simulink model "gm_uz_pmsm_model_9ph_vnl"  (R2021b)
settings: Solver=FixedStepAuto  StartTime=0.0  StopTime=0.8  RelTol=1e-3
PreLoadFcn:
  | uz_pmsm_model_9ph_init_parameter
undefined symbols (not defined in the file or in its folder): a, b, c, friction_coefficient, inertia, k_i_d, k_i_q, k_p_d, k_p_q, Kpd, L_d, L_o1, L_o2, L_q, L_x1, L_x2, L_y1, L_y2, L_zero, polepair, psi_pm, R_1, static_friction_torque, Tnd, ts
libraries: hdlmdlgenlib x191, hdlsllib x90, dspsigops x19, simulink x17, slpidlib x2, spsAlphaBetaZerotodq0Lib x1, pid_lib x1, spsdq0toAlphaBetaZeroLib x1
(part 7 of 7)

== system gm_uz_pmsm_model_9ph_vnl/uz_pmsm_model_9ph/Transformation1/Divide ==
  In1 : Inport
  In2 : Inport  Port=2
  Divide : Product  Inputs=**  OutDataTypeStr=single  SampleTime=1e-08
  Divide_pd1 : Delay  DelayLength=6
  Out1 : Outport
  wires:
  Divide_pd1/1 -> Out1/1
  Divide/1 -> Divide_pd1/1
  In2/1 -> Divide/2
  In1/1 -> Divide/1

== system gm_uz_pmsm_model_9ph_vnl/uz_pmsm_model_9ph/Transformation1/Divide1 ==
  In1 : Inport
  In2 : Inport  Port=2
  Divide1 : Product  Inputs=**  OutDataTypeStr=single  SampleTime=1e-08
  Divide1_pd1 : Delay  DelayLength=6
  Out1 : Outport
  wires:
  Divide1_pd1/1 -> Out1/1
  Divide1/1 -> Divide1_pd1/1
  In2/1 -> Divide1/2
  In1/1 -> Divide1/1

== system gm_uz_pmsm_model_9ph_vnl/uz_pmsm_model_9ph/Transformation1/Divide2 ==
  In1 : Inport
  In2 : Inport  Port=2
  Divide2 : Product  Inputs=**  OutDataTypeStr=single  SampleTime=1e-08
  Divide2_pd1 : Delay  DelayLength=6
  Out1 : Outport
  wires:
  Divide2_pd1/1 -> Out1/1
  Divide2/1 -> Divide2_pd1/1
  In2/1 -> Divide2/2
  In1/1 -> Divide2/1

== system gm_uz_pmsm_model_9ph_vnl/uz_pmsm_model_9ph/Transformation1/Divide3 ==
  In1 : Inport
  In2 : Inport  Port=2
  Divide3 : Product  Inputs=**  OutDataTypeStr=single  SampleTime=1e-08
  Divide3_pd1 : Delay  DelayLength=6
  Out1 : Outport
  wires:
  Divide3_pd1/1 -> Out1/1
  Divide3/1 -> Divide3_pd1/1
  In2/1 -> Divide3/2
  In1/1 -> Divide3/1

== system gm_uz_pmsm_model_9ph_vnl/uz_pmsm_model_9ph/Transformation1/Transformation1_MAC ==
  in0 : Inport  OutDataTypeStr=fixdt(1, 18, 16)  PortDimensions=[9 1]  SampleTime=1e-08
  in1 : Inport  Port=2  OutDataTypeStr=fixdt(1, 25, 12)  PortDimensions=[9]  SampleTime=1e-08
  globalSchedule : EnablePort  OutDataTypeStr=boolean
  PipelineRegister : Delay  DelayLength=double(8)  InitialCondition=0
  t : hdlsllib/HDL Operations/Multiply-Accumulate  opMode=Vector  initValueSetting=Dialog  initValue=0  initValueSetting2=Dialog  initValue2=0  initValueSetting3=Dialog  initValue3=0  num_samples=2  RndMeth2=Floor  RndMeth3=Floor  OutDataTypeStr=fixdt(1, 43, 28)  datatype2=Inherit: Inherit via back propagation  datatype3=Inherit: Inherit via back propagation  validOut=on  endInandOut=on  startOut=on  countOut=on  dim=-1  DoSatur=off  parallel=off
      settings: SourceProductBaseCode=SL
  out0 : Outport  OutDataTypeStr=fixdt(1, 43, 28)  SampleTime=1e-08  InitialOutput=0
  wires:
  t/1 -> PipelineRegister/1
  in1/1 -> t/2
  in0/1 -> t/1
  PipelineRegister/1 -> out0/1

== system gm_uz_pmsm_model_9ph_vnl/uz_pmsm_model_9ph/Transformation1/Transformation1_MAC1 ==
  in0 : Inport  OutDataTypeStr=fixdt(1, 18, 16)  PortDimensions=[9 1]  SampleTime=1e-08
  in1 : Inport  Port=2  OutDataTypeStr=fixdt(1, 25, 12)  PortDimensions=[9]  SampleTime=1e-08
  globalSchedule : EnablePort  OutDataTypeStr=boolean
  PipelineRegister : Delay  DelayLength=double(8)  InitialCondition=0
  t : hdlsllib/HDL Operations/Multiply-Accumulate  opMode=Vector  initValueSetting=Dialog  initValue=0  initValueSetting2=Dialog  initValue2=0  initValueSetting3=Dialog  initValue3=0  num_samples=2  RndMeth2=Floor  RndMeth3=Floor  OutDataTypeStr=fixdt(1, 43, 28)  datatype2=Inherit: Inherit via back propagation  datatype3=Inherit: Inherit via back propagation  validOut=on  endInandOut=on  startOut=on  countOut=on  dim=-1  DoSatur=off  parallel=off
      settings: SourceProductBaseCode=SL
  out0 : Outport  OutDataTypeStr=fixdt(1, 43, 28)  SampleTime=1e-08  InitialOutput=0
  wires:
  t/1 -> PipelineRegister/1
  in1/1 -> t/2
  in0/1 -> t/1
  PipelineRegister/1 -> out0/1

== system gm_uz_pmsm_model_9ph_vnl/uz_pmsm_model_9ph/Transformation1/Transformation1_MAC2 ==
  in0 : Inport  OutDataTypeStr=fixdt(1, 18, 16)  PortDimensions=[9 1]  SampleTime=1e-08
  in1 : Inport  Port=2  OutDataTypeStr=fixdt(1, 25, 12)  PortDimensions=[9]  SampleTime=1e-08
  globalSchedule : EnablePort  OutDataTypeStr=boolean
  PipelineRegister : Delay  DelayLength=double(8)  InitialCondition=0
  t : hdlsllib/HDL Operations/Multiply-Accumulate  opMode=Vector  initValueSetting=Dialog  initValue=0  initValueSetting2=Dialog  initValue2=0  initValueSetting3=Dialog  initValue3=0  num_samples=2  RndMeth2=Floor  RndMeth3=Floor  OutDataTypeStr=fixdt(1, 43, 28)  datatype2=Inherit: Inherit via back propagation  datatype3=Inherit: Inherit via back propagation  validOut=on  endInandOut=on  startOut=on  countOut=on  dim=-1  DoSatur=off  parallel=off
      settings: SourceProductBaseCode=SL
  out0 : Outport  OutDataTypeStr=fixdt(1, 43, 28)  SampleTime=1e-08  InitialOutput=0
  wires:
  t/1 -> PipelineRegister/1
  in1/1 -> t/2
  in0/1 -> t/1
  PipelineRegister/1 -> out0/1

== system gm_uz_pmsm_model_9ph_vnl/uz_pmsm_model_9ph/Transformation1/Transformation1_MAC3 ==
  in0 : Inport  OutDataTypeStr=fixdt(1, 18, 16)  PortDimensions=[9 1]  SampleTime=1e-08
  in1 : Inport  Port=2  OutDataTypeStr=fixdt(1, 25, 12)  PortDimensions=[9]  SampleTime=1e-08
  globalSchedule : EnablePort  OutDataTypeStr=boolean
  PipelineRegister : Delay  DelayLength=double(8)  InitialCondition=0
  t : hdlsllib/HDL Operations/Multiply-Accumulate  opMode=Vector  initValueSetting=Dialog  initValue=0  initValueSetting2=Dialog  initValue2=0  initValueSetting3=Dialog  initValue3=0  num_samples=2  RndMeth2=Floor  RndMeth3=Floor  OutDataTypeStr=fixdt(1, 43, 28)  datatype2=Inherit: Inherit via back propagation  datatype3=Inherit: Inherit via back propagation  validOut=on  endInandOut=on  startOut=on  countOut=on  dim=-1  DoSatur=off  parallel=off
      settings: SourceProductBaseCode=SL
  out0 : Outport  OutDataTypeStr=fixdt(1, 43, 28)  SampleTime=1e-08  InitialOutput=0
  wires:
  t/1 -> PipelineRegister/1
  in1/1 -> t/2
  in0/1 -> t/1
  PipelineRegister/1 -> out0/1

== system gm_uz_pmsm_model_9ph_vnl/uz_pmsm_model_9ph/Transformation1/Transformation1_MAC4 ==
  in0 : Inport  OutDataTypeStr=fixdt(1, 18, 16)  PortDimensions=[9 1]  SampleTime=1e-08
  in1 : Inport  Port=2  OutDataTypeStr=fixdt(1, 25, 12)  PortDimensions=[9]  SampleTime=1e-08
  globalSchedule : EnablePort  OutDataTypeStr=boolean
  PipelineRegister : Delay  DelayLength=double(8)  InitialCondition=0
  t : hdlsllib/HDL Operations/Multiply-Accumulate  opMode=Vector  initValueSetting=Dialog  initValue=0  initValueSetting2=Dialog  initValue2=0  initValueSetting3=Dialog  initValue3=0  num_samples=2  RndMeth2=Floor  RndMeth3=Floor  OutDataTypeStr=fixdt(1, 43, 28)  datatype2=Inherit: Inherit via back propagation  datatype3=Inherit: Inherit via back propagation  validOut=on  endInandOut=on  startOut=on  countOut=on  dim=-1  DoSatur=off  parallel=off
      settings: SourceProductBaseCode=SL
  out0 : Outport  OutDataTypeStr=fixdt(1, 43, 28)  SampleTime=1e-08  InitialOutput=0
  wires:
  t/1 -> PipelineRegister/1
  in1/1 -> t/2
  in0/1 -> t/1
  PipelineRegister/1 -> out0/1

== system gm_uz_pmsm_model_9ph_vnl/uz_pmsm_model_9ph/Transformation1/Transformation1_MAC5 ==
  in0 : Inport  OutDataTypeStr=fixdt(1, 18, 16)  PortDimensions=[9 1]  SampleTime=1e-08
  in1 : Inport  Port=2  OutDataTypeStr=fixdt(1, 25, 12)  PortDimensions=[9]  SampleTime=1e-08
  globalSchedule : EnablePort  OutDataTypeStr=boolean
  PipelineRegister : Delay  DelayLength=double(8)  InitialCondition=0
  t : hdlsllib/HDL Operations/Multiply-Accumulate  opMode=Vector  initValueSetting=Dialog  initValue=0  initValueSetting2=Dialog  initValue2=0  initValueSetting3=Dialog  initValue3=0  num_samples=2  RndMeth2=Floor  RndMeth3=Floor  OutDataTypeStr=fixdt(1, 43, 28)  datatype2=Inherit: Inherit via back propagation  datatype3=Inherit: Inherit via back propagation  validOut=on  endInandOut=on  startOut=on  countOut=on  dim=-1  DoSatur=off  parallel=off
      settings: SourceProductBaseCode=SL
  out0 : Outport  OutDataTypeStr=fixdt(1, 43, 28)  SampleTime=1e-08  InitialOutput=0
  wires:
  t/1 -> PipelineRegister/1
  in1/1 -> t/2
  in0/1 -> t/1
  PipelineRegister/1 -> out0/1

== system gm_uz_pmsm_model_9ph_vnl/uz_pmsm_model_9ph/Transformation1/Transformation1_MAC6 ==
  in0 : Inport  OutDataTypeStr=fixdt(1, 18, 16)  PortDimensions=[9 1]  SampleTime=1e-08
  in1 : Inport  Port=2  OutDataTypeStr=fixdt(1, 25, 12)  PortDimensions=[9]  SampleTime=1e-08
  globalSchedule : EnablePort  OutDataTypeStr=boolean
  PipelineRegister : Delay  DelayLength=double(8)  InitialCondition=0
  t : hdlsllib/HDL Operations/Multiply-Accumulate  opMode=Vector  initValueSetting=Dialog  initValue=0  initValueSetting2=Dialog  initValue2=0  initValueSetting3=Dialog  initValue3=0  num_samples=2  RndMeth2=Floor  RndMeth3=Floor  OutDataTypeStr=fixdt(1, 43, 28)  datatype2=Inherit: Inherit via back propagation  datatype3=Inherit: Inherit via back propagation  validOut=on  endInandOut=on  startOut=on  countOut=on  dim=-1  DoSatur=off  parallel=off
      settings: SourceProductBaseCode=SL
  out0 : Outport  OutDataTypeStr=fixdt(1, 43, 28)  SampleTime=1e-08  InitialOutput=0
  wires:
  t/1 -> PipelineRegister/1
  in1/1 -> t/2
  in0/1 -> t/1
  PipelineRegister/1 -> out0/1

== system gm_uz_pmsm_model_9ph_vnl/uz_pmsm_model_9ph/Transformation1/Transformation1_MAC7 ==
  in0 : Inport  OutDataTypeStr=fixdt(1, 18, 16)  PortDimensions=[9 1]  SampleTime=1e-08
  in1 : Inport  Port=2  OutDataTypeStr=fixdt(1, 25, 12)  PortDimensions=[9]  SampleTime=1e-08
  globalSchedule : EnablePort  OutDataTypeStr=boolean
  PipelineRegister : Delay  DelayLength=double(8)  InitialCondition=0
  t : hdlsllib/HDL Operations/Multiply-Accumulate  opMode=Vector  initValueSetting=Dialog  initValue=0  initValueSetting2=Dialog  initValue2=0  initValueSetting3=Dialog  initValue3=0  num_samples=2  RndMeth2=Floor  RndMeth3=Floor  OutDataTypeStr=fixdt(1, 43, 28)  datatype2=Inherit: Inherit via back propagation  datatype3=Inherit: Inherit via back propagation  validOut=on  endInandOut=on  startOut=on  countOut=on  dim=-1  DoSatur=off  parallel=off
      settings: SourceProductBaseCode=SL
  out0 : Outport  OutDataTypeStr=fixdt(1, 43, 28)  SampleTime=1e-08  InitialOutput=0
  wires:
  t/1 -> PipelineRegister/1
  in1/1 -> t/2
  in0/1 -> t/1
  PipelineRegister/1 -> out0/1

== system gm_uz_pmsm_model_9ph_vnl/uz_pmsm_model_9ph/Transformation1/Transformation1_MAC8 ==
  in0 : Inport  OutDataTypeStr=fixdt(1, 18, 16)  PortDimensions=[9 1]  SampleTime=1e-08
  in1 : Inport  Port=2  OutDataTypeStr=fixdt(1, 25, 12)  PortDimensions=[9]  SampleTime=1e-08
  globalSchedule : EnablePort  OutDataTypeStr=boolean
  PipelineRegister : Delay  DelayLength=double(8)  InitialCondition=0
  t : hdlsllib/HDL Operations/Multiply-Accumulate  opMode=Vector  initValueSetting=Dialog  initValue=0  initValueSetting2=Dialog  initValue2=0  initValueSetting3=Dialog  initValue3=0  num_samples=2  RndMeth2=Floor  RndMeth3=Floor  OutDataTypeStr=fixdt(1, 43, 28)  datatype2=Inherit: Inherit via back propagation  datatype3=Inherit: Inherit via back propagation  validOut=on  endInandOut=on  startOut=on  countOut=on  dim=-1  DoSatur=off  parallel=off
      settings: SourceProductBaseCode=SL
  out0 : Outport  OutDataTypeStr=fixdt(1, 43, 28)  SampleTime=1e-08  InitialOutput=0
  wires:
  t/1 -> PipelineRegister/1
  in1/1 -> t/2
  in0/1 -> t/1
  PipelineRegister/1 -> out0/1

== system gm_uz_pmsm_model_9ph_vnl/uz_pmsm_model_9ph/Transformation1/t3 ==
  in0 : Inport
  ColVec1 : Selector  NumberOfDimensions=2  IndexOptions=Select all,Index vector (dialog)  Indices=1,1  OutputSizes=1,1
  ColVec2 : Selector  NumberOfDimensions=2  IndexOptions=Select all,Index vector (dialog)  Indices=1,2  OutputSizes=1,1
  ColVec3 : Selector  NumberOfDimensions=2  IndexOptions=Select all,Index vector (dialog)  Indices=1,3  OutputSizes=1,1
  ColVec4 : Selector  NumberOfDimensions=2  IndexOptions=Select all,Index vector (dialog)  Indices=1,4  OutputSizes=1,1
  ColVec5 : Selector  NumberOfDimensions=2  IndexOptions=Select all,Index vector (dialog)  Indices=1,5  OutputSizes=1,1
  ColVec6 : Selector  NumberOfDimensions=2  IndexOptions=Select all,Index vector (dialog)  Indices=1,6  OutputSizes=1,1
  ColVec7 : Selector  NumberOfDimensions=2  IndexOptions=Select all,Index vector (dialog)  Indices=1,7  OutputSizes=1,1
  ColVec8 : Selector  NumberOfDimensions=2  IndexOptions=Select all,Index vector (dialog)  Indices=1,8  OutputSizes=1,1
  ColVec9 : Selector  NumberOfDimensions=2  IndexOptions=Select all,Index vector (dialog)  Indices=1,9  OutputSizes=1,1
  out0 : Outport
  out1 : Outport  Port=2
  out2 : Outport  Port=3
  out3 : Outport  Port=4
  out4 : Outport  Port=5
  out5 : Outport  Port=6
  out6 : Outport  Port=7
  out7 : Outport  Port=8
  out8 : Outport  Port=9
  wires:
  ColVec9/1 -> out8/1
  ColVec8/1 -> out7/1
  ColVec7/1 -> out6/1
  ColVec6/1 -> out5/1
  ColVec5/1 -> out4/1
  ColVec4/1 -> out3/1
  ColVec3/1 -> out2/1
  ColVec2/1 -> out1/1
  ColVec1/1 -> out0/1
  in0/1 -> ColVec9/1, ColVec8/1, ColVec7/1, ColVec6/1, ColVec5/1, ColVec4/1, ColVec3/1, ColVec2/1, ColVec1/1

== system gm_uz_pmsm_model_9ph_vnl/uz_pmsm_model_9ph/Wrapped State DTI/Compare To Constant1_relop ==
  In1 : Inport
  In2 : Inport  Port=2
  Compare To Constant1_relop : RelationalOperator  Operator=<  OutDataTypeStr=boolean  SampleTime=1e-08  RndMeth=Nearest  InputSameDT=on
  Compare To Constant1_relop_pd1 : Delay  DelayLength=1
  Out1 : Outport
  wires:
  Compare To Constant1_relop_pd1/1 -> Out1/1
  Compare To Constant1_relop/1 -> Compare To Constant1_relop_pd1/1
  In2/1 -> Compare To Constant1_relop/2
  In1/1 -> Compare To Constant1_relop/1

== system gm_uz_pmsm_model_9ph_vnl/uz_pmsm_model_9ph/Wrapped State DTI/Compare To Constant_relop ==
  In1 : Inport
  In2 : Inport  Port=2
  Compare To Constant_relop : RelationalOperator  OutDataTypeStr=boolean  SampleTime=1e-08  RndMeth=Nearest  InputSameDT=on
  Compare To Constant_relop_pd1 : Delay  DelayLength=1
  Out1 : Outport
  wires:
  Compare To Constant_relop_pd1/1 -> Out1/1
  Compare To Constant_relop/1 -> Compare To Constant_relop_pd1/1
  In2/1 -> Compare To Constant_relop/2
  In1/1 -> Compare To Constant_relop/1

== system gm_uz_pmsm_model_9ph_vnl/uz_pmsm_model_9ph/Wrapped State DTI/Gain ==
  In1 : Inport
  In2 : Inport  Port=2
  Gain : Product  Inputs=**  OutDataTypeStr=single  SampleTime=1e-08
  Gain_pd1 : Delay  DelayLength=6
  Out1 : Outport
  wires:
  Gain_pd1/1 -> Out1/1
  Gain/1 -> Gain_pd1/1
  In2/1 -> Gain/2
  In1/1 -> Gain/1

== system gm_uz_pmsm_model_9ph_vnl/uz_pmsm_model_9ph/Wrapped State DTI/Product ==
  In1 : Inport
  In2 : Inport  Port=2
  Product : Product  Inputs=**  OutDataTypeStr=single  SampleTime=1e-08
  Product_pd1 : Delay  DelayLength=6
  Out1 : Outport
  wires:
  Product_pd1/1 -> Out1/1
  Product/1 -> Product_pd1/1
  In2/1 -> Product/2
  In1/1 -> Product/1

== system gm_uz_pmsm_model_9ph_vnl/uz_pmsm_model_9ph/Wrapped State DTI/Sum ==
  In1 : Inport
  In2 : Inport  Port=2
  Sum : Sum  OutDataTypeStr=single  SampleTime=1e-08
  Sum_pd1 : Delay  DelayLength=6
  Out1 : Outport
  wires:
  Sum_pd1/1 -> Out1/1
  Sum/1 -> Sum_pd1/1
  In2/1 -> Sum/2
  In1/1 -> Sum/1

== system gm_uz_pmsm_model_9ph_vnl/uz_pmsm_model_9ph/Wrapped State DTI/Sum1 ==
  In1 : Inport
  In2 : Inport  Port=2
  Sum1 : Sum  Inputs=+-  OutDataTypeStr=single  SampleTime=1e-08
  Sum1_pd1 : Delay  DelayLength=6
  Out1 : Outport
  wires:
  Sum1_pd1/1 -> Out1/1
  Sum1/1 -> Sum1_pd1/1
  In2/1 -> Sum1/2
  In1/1 -> Sum1/1

== system gm_uz_pmsm_model_9ph_vnl/uz_pmsm_model_9ph/Wrapped State DTI/Sum2 ==
  In1 : Inport
  In2 : Inport  Port=2
  Sum2 : Sum  OutDataTypeStr=single  SampleTime=1e-08
  Sum2_pd1 : Delay  DelayLength=6
  Out1 : Outport
  wires:
  Sum2_pd1/1 -> Out1/1
  Sum2/1 -> Sum2_pd1/1
  In2/1 -> Sum2/2
  In1/1 -> Sum2/1

== system gm_uz_pmsm_model_9ph_vnl/uz_pmsm_model_9ph_vnl/Line-Line to Phase voltage/abc   to   alpha_beta_0 ==
  "a, b, c" : Inport  PortDimensions=3
  Gain2 : Gain  Gain=2/3  SaturateOnIntegerOverflow=on  OutDataTypeStr=Inherit: Same as input  ParamDataTypeStr=Inherit: Same as input
  Gain4 : Gain  Gain="[ 1   -0.5   -0.5; 0   0.5*sqrt(3)   -0.5*sqrt(3); 0.5  0.5  0.5 ]"  Multiplication=Matrix(K*u) (u vector)  SaturateOnIntegerOverflow=on  OutDataTypeStr=Inherit: Same as input  ParamDataTypeStr=Inherit: Same as input
  "alpha, beta, 0 " : Outport
  wires:
  Gain4/1 -> Gain2/1
  "a, b, c"/1 -> Gain4/1
  Gain2/1 -> "alpha, beta, 0 "/1

== system gm_uz_pmsm_model_9ph_vnl/uz_pmsm_model_9ph_vnl/Line-Line to Phase voltage/alpha_beta_0   to   abc ==
  "alpha, beta, 0  " : Inport  PortDimensions=3
  Gain4 : Gain  Gain="[ 1 0 1; -0.5   0.5*sqrt(3)  1; -0.5 -0.5*sqrt(3) 1 ]"  Multiplication=Matrix(K*u) (u vector)  SaturateOnIntegerOverflow=on  OutDataTypeStr=Inherit: Same as input  ParamDataTypeStr=Inherit: Same as input
  "a, b, c" : Outport
  wires:
  "alpha, beta, 0  "/1 -> Gain4/1
  Gain4/1 -> "a, b, c"/1

== system gm_uz_pmsm_model_9ph_vnl/uz_pmsm_model_9ph_vnl/Line-Line to Phase voltage1/abc   to   alpha_beta_0 ==
  "a, b, c" : Inport  PortDimensions=3
  Gain2 : Gain  Gain=2/3  SaturateOnIntegerOverflow=on  OutDataTypeStr=Inherit: Same as input  ParamDataTypeStr=Inherit: Same as input
  Gain4 : Gain  Gain="[ 1   -0.5   -0.5; 0   0.5*sqrt(3)   -0.5*sqrt(3); 0.5  0.5  0.5 ]"  Multiplication=Matrix(K*u) (u vector)  SaturateOnIntegerOverflow=on  OutDataTypeStr=Inherit: Same as input  ParamDataTypeStr=Inherit: Same as input
  "alpha, beta, 0 " : Outport
  wires:
  Gain2/1 -> "alpha, beta, 0 "/1
  "a, b, c"/1 -> Gain4/1
  Gain4/1 -> Gain2/1

== system gm_uz_pmsm_model_9ph_vnl/uz_pmsm_model_9ph_vnl/Line-Line to Phase voltage1/alpha_beta_0   to   abc ==
  "alpha, beta, 0  " : Inport  PortDimensions=3
  Gain4 : Gain  Gain="[ 1 0 1; -0.5   0.5*sqrt(3)  1; -0.5 -0.5*sqrt(3) 1 ]"  Multiplication=Matrix(K*u) (u vector)  SaturateOnIntegerOverflow=on  OutDataTypeStr=Inherit: Same as input  ParamDataTypeStr=Inherit: Same as input
  "a, b, c" : Outport
  wires:
  Gain4/1 -> "a, b, c"/1
  "alpha, beta, 0  "/1 -> Gain4/1

== system gm_uz_pmsm_model_9ph_vnl/uz_pmsm_model_9ph_vnl/Line-Line to Phase voltage2/abc   to   alpha_beta_0 ==
  "a, b, c" : Inport  PortDimensions=3
  Gain2 : Gain  Gain=2/3  SaturateOnIntegerOverflow=on  OutDataTypeStr=Inherit: Same as input  ParamDataTypeStr=Inherit: Same as input
  Gain4 : Gain  Gain="[ 1   -0.5   -0.5; 0   0.5*sqrt(3)   -0.5*sqrt(3); 0.5  0.5  0.5 ]"  Multiplication=Matrix(K*u) (u vector)  SaturateOnIntegerOverflow=on  OutDataTypeStr=Inherit: Same as input  ParamDataTypeStr=Inherit: Same as input
  "alpha, beta, 0 " : Outport
  wires:
  Gain4/1 -> Gain2/1
  "a, b, c"/1 -> Gain4/1
  Gain2/1 -> "alpha, beta, 0 "/1

== system gm_uz_pmsm_model_9ph_vnl/uz_pmsm_model_9ph_vnl/Line-Line to Phase voltage2/alpha_beta_0   to   abc ==
  "alpha, beta, 0  " : Inport  PortDimensions=3
  Gain4 : Gain  Gain="[ 1 0 1; -0.5   0.5*sqrt(3)  1; -0.5 -0.5*sqrt(3) 1 ]"  Multiplication=Matrix(K*u) (u vector)  SaturateOnIntegerOverflow=on  OutDataTypeStr=Inherit: Same as input  ParamDataTypeStr=Inherit: Same as input
  "a, b, c" : Outport
  wires:
  "alpha, beta, 0  "/1 -> Gain4/1
  Gain4/1 -> "a, b, c"/1

== system gm_uz_pmsm_model_9ph_vnl/uz_pmsm_model_9ph_vnl/mechanical_system/integrator ==
  in : Inport
  reset : Inport  Port=2
  Delay1 : Delay  DelayLength=1  ExternalReset=Level
      settings: InputPortMap=u0,r5
  Gain : Gain  Gain=ts  OutDataTypeStr=Inherit: Same as input
  Sum3 : Sum  Inputs=|++  OutDataTypeStr=Inherit: Same as first input
  outt : Outport
  wires:
  Sum3/1 -> Delay1/1
  Delay1/1 -> Sum3/2, outt/1
  in/1 -> Gain/1
  Gain/1 -> Sum3/1
  reset/1 -> Delay1/2

== system gm_uz_pmsm_model_9ph_vnl/uz_pmsm_model_9ph_vnl/pmsm/integrator ==
  in : Inport
  reset : Inport  Port=2
  Delay1 : Delay  DelayLength=1  ExternalReset=Level
      settings: InputPortMap=u0,r5
  Gain : Gain  Gain=ts  OutDataTypeStr=Inherit: Same as input
  Sum3 : Sum  Inputs=|++  OutDataTypeStr=Inherit: Same as first input
  outt : Outport
  wires:
  Sum3/1 -> Delay1/1
  Delay1/1 -> Sum3/2, outt/1
  in/1 -> Gain/1
  Gain/1 -> Sum3/1
  reset/1 -> Delay1/2

== system gm_uz_pmsm_model_9ph_vnl/uz_pmsm_model_9ph_vnl/pmsm/integrator1 ==
  in : Inport
  reset : Inport  Port=2
  Delay1 : Delay  DelayLength=1  ExternalReset=Level
      settings: InputPortMap=u0,r5
  Gain : Gain  Gain=ts  OutDataTypeStr=Inherit: Same as input
  Sum3 : Sum  Inputs=|++  OutDataTypeStr=Inherit: Same as first input
  outt : Outport
  wires:
  Sum3/1 -> Delay1/1
  Delay1/1 -> Sum3/2, outt/1
  in/1 -> Gain/1
  Gain/1 -> Sum3/1
  reset/1 -> Delay1/2

== system gm_uz_pmsm_model_9ph_vnl/uz_pmsm_model_9ph_vnl/pmsm/integrator2 ==
  in : Inport
  reset : Inport  Port=2
  Delay1 : Delay  DelayLength=1  ExternalReset=Level
      settings: InputPortMap=u0,r5
  Gain : Gain  Gain=ts  OutDataTypeStr=Inherit: Same as input
  Sum3 : Sum  Inputs=|++  OutDataTypeStr=Inherit: Same as first input
  outt : Outport
  wires:
  Sum3/1 -> Delay1/1
  Delay1/1 -> Sum3/2, outt/1
  in/1 -> Gain/1
  Gain/1 -> Sum3/1
  reset/1 -> Delay1/2

== system gm_uz_pmsm_model_9ph_vnl/uz_pmsm_model_9ph_vnl/pmsm/integrator3 ==
  in : Inport
  reset : Inport  Port=2
  Delay1 : Delay  DelayLength=1  ExternalReset=Level
      settings: InputPortMap=u0,r5
  Gain : Gain  Gain=ts  OutDataTypeStr=Inherit: Same as input
  Sum3 : Sum  Inputs=|++  OutDataTypeStr=Inherit: Same as first input
  outt : Outport
  wires:
  Sum3/1 -> Delay1/1
  Delay1/1 -> Sum3/2, outt/1
  in/1 -> Gain/1
  Gain/1 -> Sum3/1
  reset/1 -> Delay1/2

== system gm_uz_pmsm_model_9ph_vnl/uz_pmsm_model_9ph_vnl/pmsm/integrator4 ==
  in : Inport
  reset : Inport  Port=2
  Delay1 : Delay  DelayLength=1  ExternalReset=Level
      settings: InputPortMap=u0,r5
  Gain : Gain  Gain=ts  OutDataTypeStr=Inherit: Same as input
  Sum3 : Sum  Inputs=|++  OutDataTypeStr=Inherit: Same as first input
  outt : Outport
  wires:
  Sum3/1 -> Delay1/1
  Delay1/1 -> Sum3/2, outt/1
  in/1 -> Gain/1
  Gain/1 -> Sum3/1
  reset/1 -> Delay1/2

== system gm_uz_pmsm_model_9ph_vnl/uz_pmsm_model_9ph_vnl/pmsm/integrator5 ==
  in : Inport
  reset : Inport  Port=2
  Delay1 : Delay  DelayLength=1  ExternalReset=Level
      settings: InputPortMap=u0,r5
  Gain : Gain  Gain=ts  OutDataTypeStr=Inherit: Same as input
  Sum3 : Sum  Inputs=|++  OutDataTypeStr=Inherit: Same as first input
  outt : Outport
  wires:
  Sum3/1 -> Delay1/1
  Delay1/1 -> Sum3/2, outt/1
  in/1 -> Gain/1
  Gain/1 -> Sum3/1
  reset/1 -> Delay1/2

== system gm_uz_pmsm_model_9ph_vnl/uz_pmsm_model_9ph_vnl/pmsm/integrator6 ==
  in : Inport
  reset : Inport  Port=2
  Delay1 : Delay  DelayLength=1  ExternalReset=Level
      settings: InputPortMap=u0,r5
  Gain : Gain  Gain=ts  OutDataTypeStr=Inherit: Same as input
  Sum3 : Sum  Inputs=|++  OutDataTypeStr=Inherit: Same as first input
  outt : Outport
  wires:
  Sum3/1 -> Delay1/1
  Delay1/1 -> Sum3/2, outt/1
  in/1 -> Gain/1
  Gain/1 -> Sum3/1
  reset/1 -> Delay1/2

== system gm_uz_pmsm_model_9ph_vnl/uz_pmsm_model_9ph_vnl/pmsm/integrator7 ==
  in : Inport
  reset : Inport  Port=2
  Delay1 : Delay  DelayLength=1  ExternalReset=Level
      settings: InputPortMap=u0,r5
  Gain : Gain  Gain=ts  OutDataTypeStr=Inherit: Same as input
  Sum3 : Sum  Inputs=|++  OutDataTypeStr=Inherit: Same as first input
  outt : Outport
  wires:
  Sum3/1 -> Delay1/1
  Delay1/1 -> Sum3/2, outt/1
  in/1 -> Gain/1
  Gain/1 -> Sum3/1
  reset/1 -> Delay1/2

== system gm_uz_pmsm_model_9ph_vnl/uz_pmsm_model_9ph_vnl/pmsm/integrator8 ==
  in : Inport
  reset : Inport  Port=2
  Delay1 : Delay  DelayLength=1  ExternalReset=Level
      settings: InputPortMap=u0,r5
  Gain : Gain  Gain=ts  OutDataTypeStr=Inherit: Same as input
  Sum3 : Sum  Inputs=|++  OutDataTypeStr=Inherit: Same as first input
  outt : Outport
  wires:
  Sum3/1 -> Delay1/1
  Delay1/1 -> Sum3/2, outt/1
  in/1 -> Gain/1
  Gain/1 -> Sum3/1
  reset/1 -> Delay1/2

== system gm_uz_pmsm_model_9ph_vnl/uz_pmsm_model_9ph/Line-Line to Phase voltage/abc   to   alpha_beta_0/Gain2 ==
  In1 : Inport
  In2 : Inport  Port=2
  Gain2 : Product  Inputs=**  OutDataTypeStr=single  SaturateOnIntegerOverflow=on  SampleTime=1e-08
  Gain2_pd1 : Delay  DelayLength=6
  Out1 : Outport
  wires:
  Gain2_pd1/1 -> Out1/1
  Gain2/1 -> Gain2_pd1/1
  In2/1 -> Gain2/2
  In1/1 -> Gain2/1

== system gm_uz_pmsm_model_9ph_vnl/uz_pmsm_model_9ph/Line-Line to Phase voltage/abc   to   alpha_beta_0/MMul_add_01 ==
  In1 : Inport
  In2 : Inport  Port=2
  MMul_add_01 : Sum  OutDataTypeStr=single  SampleTime=1e-08
  MMul_add_01_pd1 : Delay  DelayLength=6
  Out1 : Outport
  wires:
  MMul_add_01_pd1/1 -> Out1/1
  MMul_add_01/1 -> MMul_add_01_pd1/1
  In2/1 -> MMul_add_01/2
  In1/1 -> MMul_add_01/1

== system gm_uz_pmsm_model_9ph_vnl/uz_pmsm_model_9ph/Line-Line to Phase voltage/abc   to   alpha_beta_0/MMul_add_12 ==
  In1 : Inport
  In2 : Inport  Port=2
  MMul_add_12 : Sum  OutDataTypeStr=single  SampleTime=1e-08
  MMul_add_12_pd1 : Delay  DelayLength=6
  Out1 : Outport
  wires:
  MMul_add_12_pd1/1 -> Out1/1
  MMul_add_12/1 -> MMul_add_12_pd1/1
  In2/1 -> MMul_add_12/2
  In1/1 -> MMul_add_12/1

== system gm_uz_pmsm_model_9ph_vnl/uz_pmsm_model_9ph/Line-Line to Phase voltage/abc   to   alpha_beta_0/MMul_dot_product ==
  In1 : Inport
  In2 : Inport  Port=2
  MMul_dot_product : Product  Inputs=**  OutDataTypeStr=single  SaturateOnIntegerOverflow=on  SampleTime=1e-08
  MMul_dot_product_pd1 : Delay  DelayLength=6
  Out1 : Outport
  wires:
  MMul_dot_product_pd1/1 -> Out1/1
  MMul_dot_product/1 -> MMul_dot_product_pd1/1
  In2/1 -> MMul_dot_product/2
  In1/1 -> MMul_dot_product/1

== system gm_uz_pmsm_model_9ph_vnl/uz_pmsm_model_9ph/Line-Line to Phase voltage/alpha_beta_0   to   abc/MMul_add_01 ==
  In1 : Inport
  In2 : Inport  Port=2
  MMul_add_01 : Sum  OutDataTypeStr=single  SampleTime=1e-08
  MMul_add_01_pd1 : Delay  DelayLength=6
  Out1 : Outport
  wires:
  MMul_add_01_pd1/1 -> Out1/1
  MMul_add_01/1 -> MMul_add_01_pd1/1
  In2/1 -> MMul_add_01/2
  In1/1 -> MMul_add_01/1

== system gm_uz_pmsm_model_9ph_vnl/uz_pmsm_model_9ph/Line-Line to Phase voltage/alpha_beta_0   to   abc/MMul_add_12 ==
  In1 : Inport
  In2 : Inport  Port=2
  MMul_add_12 : Sum  OutDataTypeStr=single  SampleTime=1e-08
  MMul_add_12_pd1 : Delay  DelayLength=6
  Out1 : Outport
  wires:
  MMul_add_12_pd1/1 -> Out1/1
  MMul_add_12/1 -> MMul_add_12_pd1/1
  In2/1 -> MMul_add_12/2
  In1/1 -> MMul_add_12/1

== system gm_uz_pmsm_model_9ph_vnl/uz_pmsm_model_9ph/Line-Line to Phase voltage/alpha_beta_0   to   abc/MMul_dot_product ==
  In1 : Inport
  In2 : Inport  Port=2
  MMul_dot_product : Product  Inputs=**  OutDataTypeStr=single  SaturateOnIntegerOverflow=on  SampleTime=1e-08
  MMul_dot_product_pd1 : Delay  DelayLength=6
  Out1 : Outport
  wires:
  MMul_dot_product_pd1/1 -> Out1/1
  MMul_dot_product/1 -> MMul_dot_product_pd1/1
  In2/1 -> MMul_dot_product/2
  In1/1 -> MMul_dot_product/1

== system gm_uz_pmsm_model_9ph_vnl/uz_pmsm_model_9ph/Line-Line to Phase voltage1/abc   to   alpha_beta_0/Gain2 ==
  In1 : Inport
  In2 : Inport  Port=2
  Gain2 : Product  Inputs=**  OutDataTypeStr=single  SaturateOnIntegerOverflow=on  SampleTime=1e-08
  Gain2_pd1 : Delay  DelayLength=6
  Out1 : Outport
  wires:
  Gain2_pd1/1 -> Out1/1
  Gain2/1 -> Gain2_pd1/1
  In2/1 -> Gain2/2
  In1/1 -> Gain2/1

== system gm_uz_pmsm_model_9ph_vnl/uz_pmsm_model_9ph/Line-Line to Phase voltage1/abc   to   alpha_beta_0/MMul_add_01 ==
  In1 : Inport
  In2 : Inport  Port=2
  MMul_add_01 : Sum  OutDataTypeStr=single  SampleTime=1e-08
  MMul_add_01_pd1 : Delay  DelayLength=6
  Out1 : Outport
  wires:
  MMul_add_01_pd1/1 -> Out1/1
  MMul_add_01/1 -> MMul_add_01_pd1/1
  In2/1 -> MMul_add_01/2
  In1/1 -> MMul_add_01/1

== system gm_uz_pmsm_model_9ph_vnl/uz_pmsm_model_9ph/Line-Line to Phase voltage1/abc   to   alpha_beta_0/MMul_add_12 ==
  In1 : Inport
  In2 : Inport  Port=2
  MMul_add_12 : Sum  OutDataTypeStr=single  SampleTime=1e-08
  MMul_add_12_pd1 : Delay  DelayLength=6
  Out1 : Outport
  wires:
  MMul_add_12_pd1/1 -> Out1/1
  MMul_add_12/1 -> MMul_add_12_pd1/1
  In2/1 -> MMul_add_12/2
  In1/1 -> MMul_add_12/1

== system gm_uz_pmsm_model_9ph_vnl/uz_pmsm_model_9ph/Line-Line to Phase voltage1/abc   to   alpha_beta_0/MMul_dot_product ==
  In1 : Inport
  In2 : Inport  Port=2
  MMul_dot_product : Product  Inputs=**  OutDataTypeStr=single  SaturateOnIntegerOverflow=on  SampleTime=1e-08
  MMul_dot_product_pd1 : Delay  DelayLength=6
  Out1 : Outport
  wires:
  MMul_dot_product_pd1/1 -> Out1/1
  MMul_dot_product/1 -> MMul_dot_product_pd1/1
  In2/1 -> MMul_dot_product/2
  In1/1 -> MMul_dot_product/1

== system gm_uz_pmsm_model_9ph_vnl/uz_pmsm_model_9ph/Line-Line to Phase voltage1/alpha_beta_0   to   abc/MMul_add_01 ==
  In1 : Inport
  In2 : Inport  Port=2
  MMul_add_01 : Sum  OutDataTypeStr=single  SampleTime=1e-08
  MMul_add_01_pd1 : Delay  DelayLength=6
  Out1 : Outport
  wires:
  MMul_add_01_pd1/1 -> Out1/1
  MMul_add_01/1 -> MMul_add_01_pd1/1
  In2/1 -> MMul_add_01/2
  In1/1 -> MMul_add_01/1

== system gm_uz_pmsm_model_9ph_vnl/uz_pmsm_model_9ph/Line-Line to Phase voltage1/alpha_beta_0   to   abc/MMul_add_12 ==
  In1 : Inport
  In2 : Inport  Port=2
  MMul_add_12 : Sum  OutDataTypeStr=single  SampleTime=1e-08
  MMul_add_12_pd1 : Delay  DelayLength=6
  Out1 : Outport
  wires:
  MMul_add_12_pd1/1 -> Out1/1
  MMul_add_12/1 -> MMul_add_12_pd1/1
  In2/1 -> MMul_add_12/2
  In1/1 -> MMul_add_12/1

== system gm_uz_pmsm_model_9ph_vnl/uz_pmsm_model_9ph/Line-Line to Phase voltage1/alpha_beta_0   to   abc/MMul_dot_product ==
  In1 : Inport
  In2 : Inport  Port=2
  MMul_dot_product : Product  Inputs=**  OutDataTypeStr=single  SaturateOnIntegerOverflow=on  SampleTime=1e-08
  MMul_dot_product_pd1 : Delay  DelayLength=6
  Out1 : Outport
  wires:
  MMul_dot_product_pd1/1 -> Out1/1
  MMul_dot_product/1 -> MMul_dot_product_pd1/1
  In2/1 -> MMul_dot_product/2
  In1/1 -> MMul_dot_product/1

== system gm_uz_pmsm_model_9ph_vnl/uz_pmsm_model_9ph/Line-Line to Phase voltage2/abc   to   alpha_beta_0/Gain2 ==
  In1 : Inport
  In2 : Inport  Port=2
  Gain2 : Product  Inputs=**  OutDataTypeStr=single  SaturateOnIntegerOverflow=on  SampleTime=1e-08
  Gain2_pd1 : Delay  DelayLength=6
  Out1 : Outport
  wires:
  Gain2_pd1/1 -> Out1/1
  Gain2/1 -> Gain2_pd1/1
  In2/1 -> Gain2/2
  In1/1 -> Gain2/1

== system gm_uz_pmsm_model_9ph_vnl/uz_pmsm_model_9ph/Line-Line to Phase voltage2/abc   to   alpha_beta_0/MMul_add_01 ==
  In1 : Inport
  In2 : Inport  Port=2
  MMul_add_01 : Sum  OutDataTypeStr=single  SampleTime=1e-08
  MMul_add_01_pd1 : Delay  DelayLength=6
  Out1 : Outport
  wires:
  MMul_add_01_pd1/1 -> Out1/1
  MMul_add_01/1 -> MMul_add_01_pd1/1
  In2/1 -> MMul_add_01/2
  In1/1 -> MMul_add_01/1

== system gm_uz_pmsm_model_9ph_vnl/uz_pmsm_model_9ph/Line-Line to Phase voltage2/abc   to   alpha_beta_0/MMul_add_12 ==
  In1 : Inport
  In2 : Inport  Port=2
  MMul_add_12 : Sum  OutDataTypeStr=single  SampleTime=1e-08
  MMul_add_12_pd1 : Delay  DelayLength=6
  Out1 : Outport
  wires:
  MMul_add_12_pd1/1 -> Out1/1
  MMul_add_12/1 -> MMul_add_12_pd1/1
  In2/1 -> MMul_add_12/2
  In1/1 -> MMul_add_12/1

== system gm_uz_pmsm_model_9ph_vnl/uz_pmsm_model_9ph/Line-Line to Phase voltage2/abc   to   alpha_beta_0/MMul_dot_product ==
  In1 : Inport
  In2 : Inport  Port=2
  MMul_dot_product : Product  Inputs=**  OutDataTypeStr=single  SaturateOnIntegerOverflow=on  SampleTime=1e-08
  MMul_dot_product_pd1 : Delay  DelayLength=6
  Out1 : Outport
  wires:
  MMul_dot_product_pd1/1 -> Out1/1
  MMul_dot_product/1 -> MMul_dot_product_pd1/1
  In2/1 -> MMul_dot_product/2
  In1/1 -> MMul_dot_product/1

== system gm_uz_pmsm_model_9ph_vnl/uz_pmsm_model_9ph/Line-Line to Phase voltage2/alpha_beta_0   to   abc/MMul_add_01 ==
  In1 : Inport
  In2 : Inport  Port=2
  MMul_add_01 : Sum  OutDataTypeStr=single  SampleTime=1e-08
  MMul_add_01_pd1 : Delay  DelayLength=6
  Out1 : Outport
  wires:
  MMul_add_01_pd1/1 -> Out1/1
  MMul_add_01/1 -> MMul_add_01_pd1/1
  In2/1 -> MMul_add_01/2
  In1/1 -> MMul_add_01/1

== system gm_uz_pmsm_model_9ph_vnl/uz_pmsm_model_9ph/Line-Line to Phase voltage2/alpha_beta_0   to   abc/MMul_add_12 ==
  In1 : Inport
  In2 : Inport  Port=2
  MMul_add_12 : Sum  OutDataTypeStr=single  SampleTime=1e-08
  MMul_add_12_pd1 : Delay  DelayLength=6
  Out1 : Outport
  wires:
  MMul_add_12_pd1/1 -> Out1/1
  MMul_add_12/1 -> MMul_add_12_pd1/1
  In2/1 -> MMul_add_12/2
  In1/1 -> MMul_add_12/1

== system gm_uz_pmsm_model_9ph_vnl/uz_pmsm_model_9ph/Line-Line to Phase voltage2/alpha_beta_0   to   abc/MMul_dot_product ==
  In1 : Inport
  In2 : Inport  Port=2
  MMul_dot_product : Product  Inputs=**  OutDataTypeStr=single  SaturateOnIntegerOverflow=on  SampleTime=1e-08
  MMul_dot_product_pd1 : Delay  DelayLength=6
  Out1 : Outport
  wires:
  MMul_dot_product_pd1/1 -> Out1/1
  MMul_dot_product/1 -> MMul_dot_product_pd1/1
  In2/1 -> MMul_dot_product/2
  In1/1 -> MMul_dot_product/1

== matlab function gm_uz_pmsm_model_9ph_vnl/Compare/Assert_outputs/RelErrCheck/RelativeErrorCheck  ==
  data: P input; y output; R input; ToleranceValue parameter double
% Check if the relative error of R with respect to P is below
% ToleranceValue
% P, R are floating-point
function y = relErrCheck(P,R, ToleranceValue)
    tol = ToleranceValue;
    sz = numel(P);
    assert(sz == numel(R), 'Inputs P and R have different sizes.');
    y = false(1, sz);

    for ii=1:sz
        if (isnan(P(ii)) || isnan(R(ii)))
            if (isnan(P(ii)) && isnan(R(ii)))
                y(ii) = true;
            end
        elseif (isinf(P(ii)) || isinf(R(ii)))
            y(ii) = (P(ii) == R(ii));
        elseif (P(ii) == 0)
            y(ii) = (R(ii) == 0);
        else
            absdiff = abs(P(ii) - R(ii));
            relerr = absdiff/abs(P(ii));
            y(ii) = (relerr <= tol);
        end
    end
end

== matlab function gm_uz_pmsm_model_9ph_vnl/Compare/Assert_i_abc_ps/RelErrCheck/RelativeErrorCheck  ==
  data: P input; y output; R input; ToleranceValue parameter double
% Check if the relative error of R with respect to P is below
% ToleranceValue
% P, R are floating-point
function y = relErrCheck(P,R, ToleranceValue)
    tol = ToleranceValue;
    sz = numel(P);
    assert(sz == numel(R), 'Inputs P and R have different sizes.');
    y = false(1, sz);

    for ii=1:sz
        if (isnan(P(ii)) || isnan(R(ii)))
            if (isnan(P(ii)) && isnan(R(ii)))
                y(ii) = true;
            end
        elseif (isinf(P(ii)) || isinf(R(ii)))
            y(ii) = (P(ii) == R(ii));
        elseif (P(ii) == 0)
            y(ii) = (R(ii) == 0);
        else
            absdiff = abs(P(ii) - R(ii));
            relerr = absdiff/abs(P(ii));
            y(ii) = (relerr <= tol);
        end
    end
end
